simulink model "Wing_Kinematics"  (R2023b)
settings: Solver=FixedStepAuto  StartTime=0.0  StopTime=5  FixedStep=dt  RelTol=1e-3
libraries: simulink_extras x1, simulink x1
settings Model: Creator=iwl  LastModifiedBy=iwl
settings ModelReferenceCC: EnableRefExpFcnMdlSchedulingChecks=on

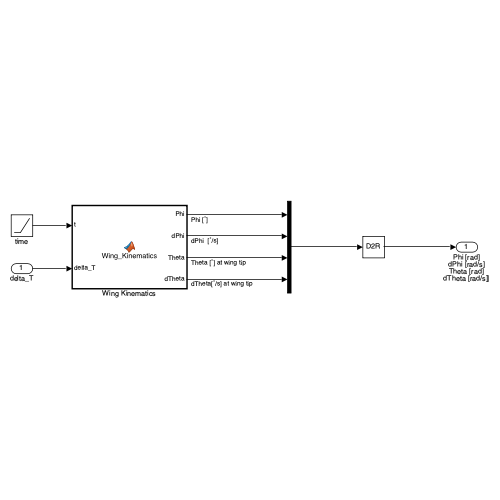
[thumbnail: Simulink's stored preview of the top-level diagram]
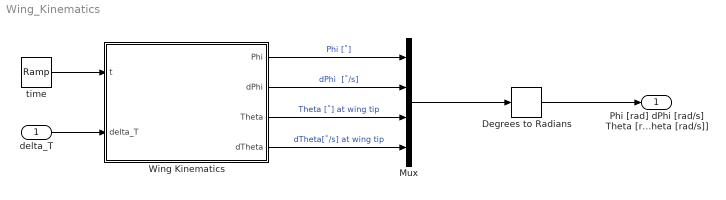
== system Wing_Kinematics ==
  delta_T : Inport
  Degrees to Radians : simulink_extras/Transformations/Degrees to Radians
  Mux : Mux
  Wing Kinematics : MATLAB Function  TreatAsAtomicUnit=on
  time : simulink/Sources/Ramp  slope=1  start=0  InitialOutput=0
  Phi [rad] dPhi [rad/s] Theta [rad] dTheta [rad/s]] : Outport
  wires:
  Wing Kinematics/3(Theta) -> Mux/3  "Theta [˚] at wing tip"
  Wing Kinematics/2(dPhi) -> Mux/2  "dPhi  [˚/s]"
  Wing Kinematics/1(Phi) -> Mux/1  "Phi [˚]"
  time/1 -> Wing Kinematics/1(t)
  Wing Kinematics/4(dTheta) -> Mux/4  "dTheta[˚/s] at wing tip"
  delta_T/1 -> Wing Kinematics/2(delta_T)
  Degrees to Radians/1 -> Phi [rad] dPhi [rad/s] Theta [rad] dTheta [rad/s]]/1
  Mux/1 -> Degrees to Radians/1

== matlab function Wing_Kinematics/Wing Kinematics ==
  data: t input; delta_T input; Phi output; Flapping parameter; dPhi output; Theta output; dTheta output
function [Phi, dPhi, Theta, dTheta] = Wing_Kinematics(t, delta_T, Flapping)
    
    f = delta_T * Flapping.f_max;                                          % [Hz]
    
    Phi  = sin(2* pi* f* t - pi/2) * Flapping.Phi_max + Flapping.Phi_off;  % [˚]

    dPhi = 2* pi* f* cos(2* pi* f* t - pi/2) * Flapping.Phi_max;           % [˚/s]

    %Theta = 0.5016 - 1.5849 * Phi - 0.0216 * dPhi, Theta as a function of Phi and dPhi
    Theta  = Flapping.Theta_max/ tanh(Flapping.K_Theta)* ...
             tanh(Flapping.K_Theta* cos(2* pi* f* t + pi/ 2));             % [˚]

    dTheta = Flapping.Theta_max/ tanh(Flapping.K_Theta)* 2* ...
             Flapping.K_Theta* f* pi* sin(pi/ 2 + 2* pi* f* t)* ...
             (tanh((Flapping.K_Theta* cos(pi/ 2 + 2* pi* f* t)))^2 - 1);   % [˚]

end
